simulink model "TAL220"  (R2020a)
settings: Solver=FixedStepAuto  StartTime=0.0  StopTime=10.0  RelTol=1e-3
values from neighbouring files (symbols this model uses):
  TAL220_load_variance = 0.001^2    (= 1e-06)    [configure_simulation.m]
  TAL220_sample_rate = 10    [configure_simulation.m]
settings Model: Creator=Philip  LastModifiedBy=Philip

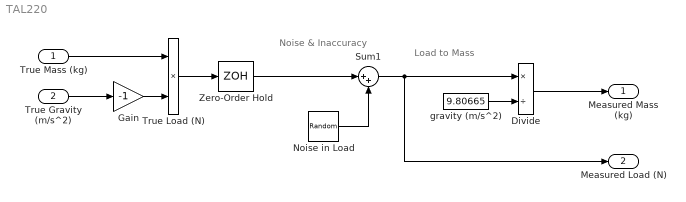
== system TAL220 ==
  note: Load to Mass
  note: Noise & Inaccuracy
  True Mass (kg) : Inport
  True Gravity (m/s^2) : Inport  Port=2
  Divide : Product  Inputs=*/
  Gain : Gain  Gain=-1
  Noise in Load : RandomNumber  Variance=TAL220_load_variance  SampleTime=1/TAL220_sample_rate
  Sum1 : Sum  Inputs=|++
  True Load (N) : Product
  Zero-Order Hold : ZeroOrderHold  SampleTime=1/TAL220_sample_rate
  gravity (m/s^2) : Constant  Value=9.80665
  Measured Mass (kg) : Outport
  Measured Load (N) : Outport  Port=2
  wires:
  True Mass (kg)/1 -> True Load (N)/1
  Noise in Load/1 -> Sum1/2
  True Load (N)/1 -> Zero-Order Hold/1
  True Gravity (m/s^2)/1 -> Gain/1
  gravity (m/s^2)/1 -> Divide/2
  Sum1/1 -> Measured Load (N)/1, Divide/1
  Divide/1 -> Measured Mass (kg)/1
  Zero-Order Hold/1 -> Sum1/1
  Gain/1 -> True Load (N)/2
